simulink model "test_direct"  (R2024a)
settings: Solver=VariableStepAuto  StartTime=0.0  StopTime=40  RelTol=1e-3
libraries: neural x733, simulink x4
(part 35 of 35)

== system test_direct/Function Fitting Neural Network6/Layer 6/Delays 1 ==
  "p{6}" : Inport  PortDimensions=20
      mask Display: e = 0.06;c1 = [120 230 180]/255;c2 = ([120 230 180]+0)/(256+128);c3 = ([120 230 180]+128)/(256+128);patch([0 1 1 0],[0 0 1 1],c1);patch([0 1 1 1-e 1-e 0+e],[0 0 1 1-e 0+e 0+e],c2);patch([0 0 1 1-e 0+e 0+e],[0 1 1 1-e 1-e 0+e],c3);plot([0 1 1 0 0],[0 0 1 1 0]);
  mux : Mux  Inputs=1
      mask Display: e = 0.06;c1 = [120 150 230]/255;c2 = ([120 150 230]+0)/383;c3 = ([120 150 230]+128)/383;patch([0 1 1 0],[0 0 1 1],c1);patch([0 1 1 1-e 1-e 0+e],[0 0 1 1-e 0+e 0+e],c2);patch([0 0 1 1-e 0+e 0+e],[0 1 1 1-e 1-e 0+e],c3);plot([0 1 1 0 0],[0 0 1 1 0]);disp('Mux')
  "pd{6,5}" : Outport
      mask Display: e = 0.06;c1 = [120 230 180]/255;c2 = ([120 230 180]+0)/(256+128);c3 = ([120 230 180]+128)/(256+128);patch([0 1 1 0],[0 0 1 1],c1);patch([0 1 1 1-e 1-e 0+e],[0 0 1 1-e 0+e 0+e],c2);patch([0 0 1 1-e 0+e 0+e],[0 1 1 1-e 1-e 0+e],c3);plot([0 1 1 0 0],[0 0 1 1 0]);
  wires:
  "p{6}"/1 -> mux/1
  mux/1 -> "pd{6,5}"/1

== system test_direct/Function Fitting Neural Network6/Layer 6/LW{6,5} ==
  "ad{6,5}" : Inport  PortDimensions=20
      mask Display: e = 0.06;c1 = [120 230 180]/255;c2 = ([120 230 180]+0)/(256+128);c3 = ([120 230 180]+128)/(256+128);patch([0 1 1 0],[0 0 1 1],c1);patch([0 1 1 1-e 1-e 0+e],[0 0 1 1-e 0+e 0+e],c2);patch([0 0 1 1-e 0+e 0+e],[0 1 1 1-e 1-e 0+e],c3);plot([0 1 1 0 0],[0 0 1 1 0]);
  "IW{6,5}(1,:)'" : Constant  Value=[0.397882150641937271107195783770293928682804107666015625;0.468082027941522371694560433752485550940036773681640625;0.295246457733882028406924291630275547504425048828125;0.455024034822306522318768884360906668007373809814453125;-0.303493600579253064442042386872344650328159332275390625;0.540067390854785056575337875983677804470062255859375;0.1123163355927400963718554294246132485568523406982421875;0.217862596811197573032359287026338279247283935546875;-0.390161183349621742966206738856271840631961822509765625;0.10197970732984795727560367595287971198558807373046875;-0.02977337885287738294959325457966770045459270477294921875;0.5629603029920684509335160328191705048084259033203125;0.00897396596046501869581302202050210325978696346282958984375;0.1735034525327801280258910310294595547020435333251953125;-0.52952282982221310358994514899677596986293792724609375;-0.405354172745957141987815930406213738024234771728515625;0.51376817545518382868152684750384651124477386474609375;0.1169943691200735214064110323306522332131862640380859375;-0.1975012009013779046284753349027596414089202880859375;0.14996823670384451521186974787269718945026397705078125]
      mask Display: e = 0.06;c1 = [120 150 230]/255;c2 = ([120 150 230]+0)/383;c3 = ([120 150 230]+128)/383;patch([0 1 1 0],[0 0 1 1],c1);patch([0 1 1 1-e 1-e 0+e],[0 0 1 1-e 0+e 0+e],c2);patch([0 0 1 1-e 0+e 0+e],[0 1 1 1-e 1-e 0+e],c3);plot([0 1 1 0 0],[0 0 1 1 0]);disp('weights');
  "IW{6,5}(10,:)'" : Constant  Value=[-0.1315178910759744468350618262775242328643798828125;-0.11570394784521360886930807509997976012527942657470703125;0.0264935027116691874937703943260203232057392597198486328125;0.23009040321696272446416742241126485168933868408203125;0.44543628656753408989743547863326966762542724609375;-0.494920438892067771075033988381619565188884735107421875;0.3542315548965608851261777090257965028285980224609375;-0.0315268050601491267581621968929539434611797332763671875;0.045284878261053491954601923907830496318638324737548828125;0.281099548637851415211486028056242503225803375244140625;0.3298637896019618320764266172773204743862152099609375;0.220315749061302523781336049069068394601345062255859375;-0.384735381199918291539319170624366961419582366943359375;0.56722214501023981991778555311611853539943695068359375;0.60882922499176606034865244510001502931118011474609375;0.440494199476847037022508857262437231838703155517578125;-0.4506550199091723385436125681735575199127197265625;0.1453933245614437985704370248640771023929119110107421875;-0.2318306587271542762440645901733660139143466949462890625;0.52564211590665166351499237862299196422100067138671875]
      mask Display: e = 0.06;c1 = [120 150 230]/255;c2 = ([120 150 230]+0)/383;c3 = ([120 150 230]+128)/383;patch([0 1 1 0],[0 0 1 1],c1);patch([0 1 1 1-e 1-e 0+e],[0 0 1 1-e 0+e 0+e],c2);patch([0 0 1 1-e 0+e 0+e],[0 1 1 1-e 1-e 0+e],c3);plot([0 1 1 0 0],[0 0 1 1 0]);disp('weights');
  "IW{6,5}(2,:)'" : Constant  Value=[-0.259863046679477072142816496125306002795696258544921875;-0.1830984540752686740017196598273585550487041473388671875;-0.40783762651549382294291490325122140347957611083984375;0.5565041642915300457161720260046422481536865234375;0.0251316487867703670933128279330048826523125171661376953125;-0.54296524298790427298655458798748441040515899658203125;0.1997883270174145853292912988763418979942798614501953125;0.314103138320985852960376405462739057838916778564453125;-0.324432365229379182647306834041955880820751190185546875;-0.1525621807993685907778314003735431469976902008056640625;0.53845616316799149725369488805881701409816741943359375;-0.250784765409623633392044439460732974112033843994140625;-0.10606220961189649631961628983845002949237823486328125;0.1157948484632281560546829268787405453622341156005859375;-0.51807744838450264790452592933434061706066131591796875;-0.6857041723316272818777861175476573407649993896484375;0.10920487886410711053652988766771159134805202484130859375;-0.313138255833295797714299624203704297542572021484375;0.38469132727216004408177241202793084084987640380859375;0.219205655925688358554026535784942097961902618408203125]
      mask Display: e = 0.06;c1 = [120 150 230]/255;c2 = ([120 150 230]+0)/383;c3 = ([120 150 230]+128)/383;patch([0 1 1 0],[0 0 1 1],c1);patch([0 1 1 1-e 1-e 0+e],[0 0 1 1-e 0+e 0+e],c2);patch([0 0 1 1-e 0+e 0+e],[0 1 1 1-e 1-e 0+e],c3);plot([0 1 1 0 0],[0 0 1 1 0]);disp('weights');
  "IW{6,5}(3,:)'" : Constant  Value=[-0.322191446388043811754897660648566670715808868408203125;0.12943750075051230208345032224315218627452850341796875;0.4237040157630704850788561088847927749156951904296875;-0.28820692308215623000933192088268697261810302734375;0.3094621696302846114434714763774536550045013427734375;-0.07740430882477371266059407162174466066062450408935546875;-0.166363695923615606542256273314706049859523773193359375;0.274876958130420623316325645646429620683193206787109375;-0.3624056774348793918960609516943804919719696044921875;0.360905335276304806146896453356021083891391754150390625;-0.035341710122767384938402557281733606941998004913330078125;0.45960431193760931112279877197579480707645416259765625;0.422640277104020245513282816318678669631481170654296875;-0.276943692378282813049139576833113096654415130615234375;0.38403391359010663475004321298911236226558685302734375;0.3141605407476737443772663027630187571048736572265625;0.5701700921924774956295323136146180331707000732421875;0.3699891159909345361711530131287872791290283203125;-0.2836815610168057499862470649532042443752288818359375;0.385139073042050916750866917936946265399456024169921875]
      mask Display: e = 0.06;c1 = [120 150 230]/255;c2 = ([120 150 230]+0)/383;c3 = ([120 150 230]+128)/383;patch([0 1 1 0],[0 0 1 1],c1);patch([0 1 1 1-e 1-e 0+e],[0 0 1 1-e 0+e 0+e],c2);patch([0 0 1 1-e 0+e 0+e],[0 1 1 1-e 1-e 0+e],c3);plot([0 1 1 0 0],[0 0 1 1 0]);disp('weights');
  "IW{6,5}(4,:)'" : Constant  Value=[-0.311849139023206711751612374428077600896358489990234375;-0.26903765327238726712266725371591746807098388671875;-0.1475542533708005255022044366342015564441680908203125;-0.00438287554053127560715896748888553702272474765777587890625;-0.470596852952205491060766462396713905036449432373046875;0.187441234110062582285394228165387175977230072021484375;-0.02028579377650745196870474273964646272361278533935546875;-0.1706606059742805658885345110320486128330230712890625;-0.263076491594098682558211521609337069094181060791015625;0.482406460346789855986315842528711073100566864013671875;-0.2397596597921014538457029630080796778202056884765625;0.5694845081120332164204000946483574807643890380859375;0.573143311906682217937714085564948618412017822265625;0.3550840700523314463765700566000305116176605224609375;-0.10464808133505164311483071060138172470033168792724609375;0.1324206560678918009887894413623143918812274932861328125;0.491379806997724155603890494603547267615795135498046875;-0.4102115364803180508346258648089133203029632568359375;0.4629653805545992373282615517382510006427764892578125;0.43274210314075889360907467562356032431125640869140625]
      mask Display: e = 0.06;c1 = [120 150 230]/255;c2 = ([120 150 230]+0)/383;c3 = ([120 150 230]+128)/383;patch([0 1 1 0],[0 0 1 1],c1);patch([0 1 1 1-e 1-e 0+e],[0 0 1 1-e 0+e 0+e],c2);patch([0 0 1 1-e 0+e 0+e],[0 1 1 1-e 1-e 0+e],c3);plot([0 1 1 0 0],[0 0 1 1 0]);disp('weights');
  "IW{6,5}(5,:)'" : Constant  Value=[0.39076466508730189897136142462841235101222991943359375;0.59687496366507819534064083200064487755298614501953125;0.60388735365921031306157829021685756742954254150390625;0.391083510505554510228165554508450441062450408935546875;0.1857553783889999976519646907036076299846172332763671875;0.058357104078057338292229161424984340555965900421142578125;0.435061422185155810549161969902343116700649261474609375;0.370616314351330411458462776863598264753818511962890625;0.0172696275587367990833609354694999638013541698455810546875;0.1838394530689289041447409545071423053741455078125;0.07328410075632295350711586934266961179673671722412109375;-0.57099991809735872738684747673687525093555450439453125;0.39539640481434312757613724897964857518672943115234375;0.01533020880475842277756992615422859671525657176971435546875;0.182469533417668194896776867608423344790935516357421875;0.0186186383865887539190708821479347534477710723876953125;0.247471549691458070352467757402337156236171722412109375;0.58505277158964397177243199621443636715412139892578125;0.0269860185739918441438778273777643335051834583282470703125;0.28827890201689354565672829266986809670925140380859375]
      mask Display: e = 0.06;c1 = [120 150 230]/255;c2 = ([120 150 230]+0)/383;c3 = ([120 150 230]+128)/383;patch([0 1 1 0],[0 0 1 1],c1);patch([0 1 1 1-e 1-e 0+e],[0 0 1 1-e 0+e 0+e],c2);patch([0 0 1 1-e 0+e 0+e],[0 1 1 1-e 1-e 0+e],c3);plot([0 1 1 0 0],[0 0 1 1 0]);disp('weights');
  "IW{6,5}(6,:)'" : Constant  Value=[-0.06774024076759577184247973491437733173370361328125;0.121240957121928005779665227237273938953876495361328125;0.00283361648694205846277238691754973842762410640716552734375;-0.5208699804879179939831601586774922907352447509765625;0.2784796701698939447311431649723090231418609619140625;-0.592047286953672813325511015136726200580596923828125;-0.1739175172878369146634014441588078625500202178955078125;0.60070560648774617984457790953456424176692962646484375;0.046111739861256433037350888071159715764224529266357421875;0.0943204616791440686451863939510076306760311126708984375;0.43961382648697477915078479782096110284328460693359375;0.11784980869757584465151722952214186079800128936767578125;-0.38960310737365322353298324742354452610015869140625;-0.11942314017125323089008048782488913275301456451416015625;-0.254362710109897582899662893396453000605106353759765625;0.5408412312419075274050328516750596463680267333984375;-0.42003913808441717403496795668615959584712982177734375;-0.1933975398610572049573619324291939847171306610107421875;-0.469061493772964854809259804824250750243663787841796875;-0.48740730169550372519182701580575667321681976318359375]
      mask Display: e = 0.06;c1 = [120 150 230]/255;c2 = ([120 150 230]+0)/383;c3 = ([120 150 230]+128)/383;patch([0 1 1 0],[0 0 1 1],c1);patch([0 1 1 1-e 1-e 0+e],[0 0 1 1-e 0+e 0+e],c2);patch([0 0 1 1-e 0+e 0+e],[0 1 1 1-e 1-e 0+e],c3);plot([0 1 1 0 0],[0 0 1 1 0]);disp('weights');
  "IW{6,5}(7,:)'" : Constant  Value=[-0.1178531446253089642883793430883088149130344390869140625;0.0256280438722267522866360422995057888329029083251953125;-0.135961816484338304800161267849034629762172698974609375;-0.290819500835572342101187359730829484760761260986328125;0.57775241023036716381255928354221396148204803466796875;0.48805729645518602932696694551850669085979461669921875;-0.50179714395470842447366521810181438922882080078125;0.56522137278847328634157065607723779976367950439453125;0.364043989376938548208073598289047367870807647705078125;0.3720816754895814870707226873491890728473663330078125;-0.00620691534365405868378662290751890395767986774444580078125;0.66496191038600682698955779414973221719264984130859375;0.09119345368104352089755337829046766273677349090576171875;-0.2028506689816634012135665443565812893211841583251953125;0.421603273778618170553045274573378264904022216796875;-0.33519033565116362893832047120667994022369384765625;-0.11053155968370820261270637274719774723052978515625;-0.2204212433030242890286132251276285387575626373291015625;-0.55861847705264555674631310466793365776538848876953125;-0.3566629493677646589588903225376270711421966552734375]
      mask Display: e = 0.06;c1 = [120 150 230]/255;c2 = ([120 150 230]+0)/383;c3 = ([120 150 230]+128)/383;patch([0 1 1 0],[0 0 1 1],c1);patch([0 1 1 1-e 1-e 0+e],[0 0 1 1-e 0+e 0+e],c2);patch([0 0 1 1-e 0+e 0+e],[0 1 1 1-e 1-e 0+e],c3);plot([0 1 1 0 0],[0 0 1 1 0]);disp('weights');
  "IW{6,5}(8,:)'" : Constant  Value=[0.3418012900238263096497348669799976050853729248046875;0.438053862441932562177271393011324107646942138671875;-0.12054184611126117498969279040466062724590301513671875;-0.546571432379943988877357696765102446079254150390625;0.654734221497687673974041899782605469226837158203125;0.430179920110494273810530785340233705937862396240234375;0.12146279436727568101783703014007187448441982269287109375;0.07559279869561878750783279201641562394797801971435546875;0.527205954397961473745226612663827836513519287109375;-0.3492582745538594934942011605016887187957763671875;0.265600306877053438103786220381152816116809844970703125;-0.2187601723385237673102921007739496417343616485595703125;0.5802937967424506293667718637152574956417083740234375;0.210866613171343530996892923212726600468158721923828125;-0.251834699178452525725191435412853024899959564208984375;0.05202462450641291702435609067833865992724895477294921875;0.279091656512666208556083802250213921070098876953125;-0.325365473340081090558584264726960100233554840087890625;-0.67999090532277473020172919859760440886020660400390625;-0.003136982141041910754353239099145866930484771728515625]
      mask Display: e = 0.06;c1 = [120 150 230]/255;c2 = ([120 150 230]+0)/383;c3 = ([120 150 230]+128)/383;patch([0 1 1 0],[0 0 1 1],c1);patch([0 1 1 1-e 1-e 0+e],[0 0 1 1-e 0+e 0+e],c2);patch([0 0 1 1-e 0+e 0+e],[0 1 1 1-e 1-e 0+e],c3);plot([0 1 1 0 0],[0 0 1 1 0]);disp('weights');
  "IW{6,5}(9,:)'" : Constant  Value=[-0.254277325057250092044114353484474122524261474609375;-0.275668684735444202704712779450346715748310089111328125;0.414659628489796094896746581071056425571441650390625;0.403068133475517509367591628688387572765350341796875;-0.1787498495362999928470770782951149158179759979248046875;-0.154238015270505235410070099533186294138431549072265625;0.018894261147071815531983673963623004965484142303466796875;0.55285835915803094309239895665086805820465087890625;-0.352382081684923520459307155761052854359149932861328125;0.52875023669751575194908355115330778062343597412109375;0.11313827261161078785445255334707326255738735198974609375;-0.083147258416225999777537936097360216081142425537109375;0.51749661983667516462759294881834648549556732177734375;-0.0452763817258667600196275770940701477229595184326171875;-0.2325122784106159468109353838372044265270233154296875;0.278746434133094134200092639730428345501422882080078125;-0.45600994524341842417669568021665327250957489013671875;0.55958105526593104883659179904498159885406494140625;0.5043075017813902771735001806518994271755218505859375;-0.1662493916690039041927917651264579035341739654541015625]
      mask Display: e = 0.06;c1 = [120 150 230]/255;c2 = ([120 150 230]+0)/383;c3 = ([120 150 230]+128)/383;patch([0 1 1 0],[0 0 1 1],c1);patch([0 1 1 1-e 1-e 0+e],[0 0 1 1-e 0+e 0+e],c2);patch([0 0 1 1-e 0+e 0+e],[0 1 1 1-e 1-e 0+e],c3);plot([0 1 1 0 0],[0 0 1 1 0]);disp('weights');
  Mux : Mux  Inputs=10
      mask Display: e = 0.06;c1 = [120 150 230]/255;c2 = ([120 150 230]+0)/383;c3 = ([120 150 230]+128)/383;patch([0 1 1 0],[0 0 1 1],c1);patch([0 1 1 1-e 1-e 0+e],[0 0 1 1-e 0+e 0+e],c2);patch([0 0 1 1-e 0+e 0+e],[0 1 1 1-e 1-e 0+e],c3);plot([0 1 1 0 0],[0 0 1 1 0]);disp('Mux');
  dotprod{1..10} (10 alike) : neural/Weight Functions/dotprod
  "lz{6,5}" : Outport
      mask Display: e = 0.06;c1 = [120 230 180]/255;c2 = ([120 230 180]+0)/(256+128);c3 = ([120 230 180]+128)/(256+128);patch([0 1 1 0],[0 0 1 1],c1);patch([0 1 1 1-e 1-e 0+e],[0 0 1 1-e 0+e 0+e],c2);patch([0 0 1 1-e 0+e 0+e],[0 1 1 1-e 1-e 0+e],c3);plot([0 1 1 0 0],[0 0 1 1 0]);
  wires:
  "IW{6,5}(1,:)'"/1 -> dotprod1/1
  "ad{6,5}"/1 -> dotprod1/2, dotprod2/2, dotprod3/2, dotprod4/2, dotprod5/2, dotprod6/2, dotprod7/2, dotprod8/2, dotprod9/2, dotprod10/2
  dotprod1/1 -> Mux/1
  "IW{6,5}(2,:)'"/1 -> dotprod2/1
  dotprod2/1 -> Mux/2
  "IW{6,5}(3,:)'"/1 -> dotprod3/1
  dotprod3/1 -> Mux/3
  "IW{6,5}(4,:)'"/1 -> dotprod4/1
  dotprod4/1 -> Mux/4
  "IW{6,5}(5,:)'"/1 -> dotprod5/1
  dotprod5/1 -> Mux/5
  "IW{6,5}(6,:)'"/1 -> dotprod6/1
  dotprod6/1 -> Mux/6
  "IW{6,5}(7,:)'"/1 -> dotprod7/1
  dotprod7/1 -> Mux/7
  "IW{6,5}(8,:)'"/1 -> dotprod8/1
  dotprod8/1 -> Mux/8
  "IW{6,5}(9,:)'"/1 -> dotprod9/1
  dotprod9/1 -> Mux/9
  "IW{6,5}(10,:)'"/1 -> dotprod10/1
  dotprod10/1 -> Mux/10
  Mux/1 -> "lz{6,5}"/1

== system test_direct/Function Fitting Neural Network6/Layer 7/Delays 1 ==
  "p{7}" : Inport  PortDimensions=10
      mask Display: e = 0.06;c1 = [120 230 180]/255;c2 = ([120 230 180]+0)/(256+128);c3 = ([120 230 180]+128)/(256+128);patch([0 1 1 0],[0 0 1 1],c1);patch([0 1 1 1-e 1-e 0+e],[0 0 1 1-e 0+e 0+e],c2);patch([0 0 1 1-e 0+e 0+e],[0 1 1 1-e 1-e 0+e],c3);plot([0 1 1 0 0],[0 0 1 1 0]);
  mux : Mux  Inputs=1
      mask Display: e = 0.06;c1 = [120 150 230]/255;c2 = ([120 150 230]+0)/383;c3 = ([120 150 230]+128)/383;patch([0 1 1 0],[0 0 1 1],c1);patch([0 1 1 1-e 1-e 0+e],[0 0 1 1-e 0+e 0+e],c2);patch([0 0 1 1-e 0+e 0+e],[0 1 1 1-e 1-e 0+e],c3);plot([0 1 1 0 0],[0 0 1 1 0]);disp('Mux')
  "pd{7,6}" : Outport
      mask Display: e = 0.06;c1 = [120 230 180]/255;c2 = ([120 230 180]+0)/(256+128);c3 = ([120 230 180]+128)/(256+128);patch([0 1 1 0],[0 0 1 1],c1);patch([0 1 1 1-e 1-e 0+e],[0 0 1 1-e 0+e 0+e],c2);patch([0 0 1 1-e 0+e 0+e],[0 1 1 1-e 1-e 0+e],c3);plot([0 1 1 0 0],[0 0 1 1 0]);
  wires:
  "p{7}"/1 -> mux/1
  mux/1 -> "pd{7,6}"/1

== system test_direct/Function Fitting Neural Network6/Layer 7/LW{7,6} ==
  "ad{7,6}" : Inport  PortDimensions=10
      mask Display: e = 0.06;c1 = [120 230 180]/255;c2 = ([120 230 180]+0)/(256+128);c3 = ([120 230 180]+128)/(256+128);patch([0 1 1 0],[0 0 1 1],c1);patch([0 1 1 1-e 1-e 0+e],[0 0 1 1-e 0+e 0+e],c2);patch([0 0 1 1-e 0+e 0+e],[0 1 1 1-e 1-e 0+e],c3);plot([0 1 1 0 0],[0 0 1 1 0]);
  "IW{7,6}(1,:)'" : Constant  Value=[-0.267007107036910718012023835399304516613483428955078125;0.1396932912003606419570900243343203328549861907958984375;0.56416598011940666257402199335047043859958648681640625;0.374390432776119108648771316438796930015087127685546875;0.72544051450457469609744975969078950583934783935546875;0.90508281455128436476798015064559876918792724609375;-1.230102223653959381266531636356376111507415771484375;-0.51314258262198197968473323271609842777252197265625;0.006260373640057360911104211709243827499449253082275390625;0.270013248873878008993187904707156121730804443359375]
      mask Display: e = 0.06;c1 = [120 150 230]/255;c2 = ([120 150 230]+0)/383;c3 = ([120 150 230]+128)/383;patch([0 1 1 0],[0 0 1 1],c1);patch([0 1 1 1-e 1-e 0+e],[0 0 1 1-e 0+e 0+e],c2);patch([0 0 1 1-e 0+e 0+e],[0 1 1 1-e 1-e 0+e],c3);plot([0 1 1 0 0],[0 0 1 1 0]);disp('weights');
  "IW{7,6}(2,:)'" : Constant  Value=[-0.1501267963351574918906550237807095982134342193603515625;-1.087754781444640883592001046054065227508544921875;0.50879152017675532970741869576158933341503143310546875;0.205766145581553761001458724422263912856578826904296875;-0.228012997535293748807561087232897989451885223388671875;-0.32415818152162756415890498828957788646221160888671875;0.2383509034293116446434623867389746010303497314453125;0.556903774080990121575496232253499329090118408203125;-0.06343658027983763159074470650011789985001087188720703125;0.446761525323581099033987129587330855429172515869140625]
      mask Display: e = 0.06;c1 = [120 150 230]/255;c2 = ([120 150 230]+0)/383;c3 = ([120 150 230]+128)/383;patch([0 1 1 0],[0 0 1 1],c1);patch([0 1 1 1-e 1-e 0+e],[0 0 1 1-e 0+e 0+e],c2);patch([0 0 1 1-e 0+e 0+e],[0 1 1 1-e 1-e 0+e],c3);plot([0 1 1 0 0],[0 0 1 1 0]);disp('weights');
  Mux : Mux  Inputs=2
      mask Display: e = 0.06;c1 = [120 150 230]/255;c2 = ([120 150 230]+0)/383;c3 = ([120 150 230]+128)/383;patch([0 1 1 0],[0 0 1 1],c1);patch([0 1 1 1-e 1-e 0+e],[0 0 1 1-e 0+e 0+e],c2);patch([0 0 1 1-e 0+e 0+e],[0 1 1 1-e 1-e 0+e],c3);plot([0 1 1 0 0],[0 0 1 1 0]);disp('Mux');
  dotprod1 : neural/Weight Functions/dotprod
  dotprod2 : neural/Weight Functions/dotprod
  "lz{7,6}" : Outport
      mask Display: e = 0.06;c1 = [120 230 180]/255;c2 = ([120 230 180]+0)/(256+128);c3 = ([120 230 180]+128)/(256+128);patch([0 1 1 0],[0 0 1 1],c1);patch([0 1 1 1-e 1-e 0+e],[0 0 1 1-e 0+e 0+e],c2);patch([0 0 1 1-e 0+e 0+e],[0 1 1 1-e 1-e 0+e],c3);plot([0 1 1 0 0],[0 0 1 1 0]);
  wires:
  "IW{7,6}(1,:)'"/1 -> dotprod1/1
  "ad{7,6}"/1 -> dotprod1/2, dotprod2/2
  dotprod1/1 -> Mux/1
  "IW{7,6}(2,:)'"/1 -> dotprod2/1
  dotprod2/1 -> Mux/2
  Mux/1 -> "lz{7,6}"/1
